simulink model "Environment"  (R2012b)
settings: Solver=FixedStepDiscrete  StartTime=0.0  StopTime=10.0  FixedStep=delta_t  RelTol=1e-3
settings Model: Creator=Kerianne  LastModifiedBy=Kerianne
settings DataIOCC: SaveFormat=Structure
settings OptimizationCC: InlineParams=on

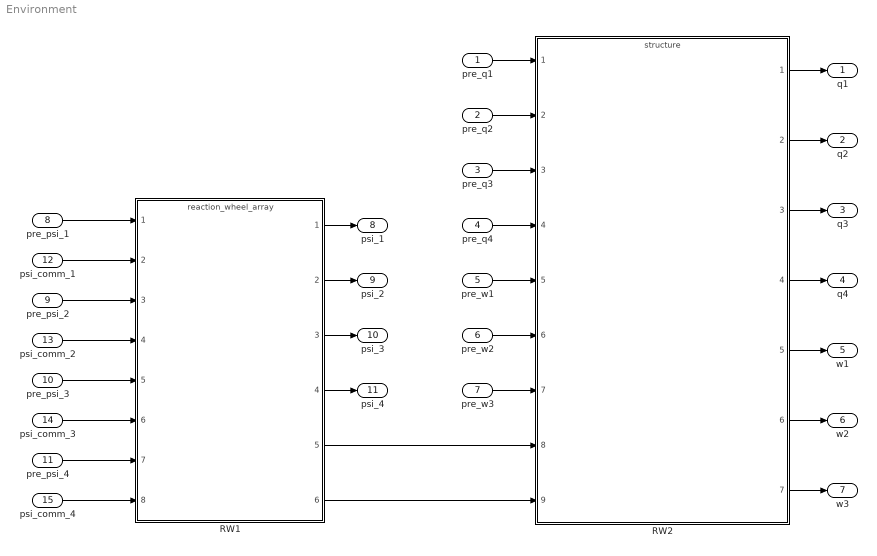
== system Environment ==
  pre_q1 : Inport
  pre_q2 : Inport  Port=2
  pre_q3 : Inport  Port=3
  pre_q4 : Inport  Port=4
  pre_w1 : Inport  Port=5
  pre_w2 : Inport  Port=6
  pre_w3 : Inport  Port=7
  pre_psi_1 : Inport  Port=8
  pre_psi_2 : Inport  Port=9
  pre_psi_3 : Inport  Port=10
  pre_psi_4 : Inport  Port=11
  "psi_comm_1 " : Inport  Port=12
  psi_comm_2 : Inport  Port=13
  psi_comm_3 : Inport  Port=14
  psi_comm_4 : Inport  Port=15
  RW1 : ModelReference  ModelNameDialog=reaction_wheel_array  SimulationMode=Normal  ModelReferenceVersion=1.14  CopyOfModelName=reaction_wheel_array  DefaultDataLogging=on
  RW2 : ModelReference  ModelNameDialog=structure  SimulationMode=Normal  ModelReferenceVersion=1.10  CopyOfModelName=structure  DefaultDataLogging=on
  q1 : Outport
  q2 : Outport  Port=2
  q3 : Outport  Port=3
  q4 : Outport  Port=4
  w1 : Outport  Port=5
  w2 : Outport  Port=6
  w3 : Outport  Port=7
  psi_1 : Outport  Port=8
  psi_2 : Outport  Port=9
  psi_3 : Outport  Port=10
  psi_4 : Outport  Port=11
  wires:
  pre_psi_1/1 -> RW1/1
  "psi_comm_1 "/1 -> RW1/2
  pre_psi_2/1 -> RW1/3
  psi_comm_2/1 -> RW1/4
  pre_psi_3/1 -> RW1/5
  psi_comm_3/1 -> RW1/6
  RW2/7 -> w3/1
  RW2/6 -> w2/1
  RW2/5 -> w1/1
  RW2/4 -> q4/1
  RW2/3 -> q3/1
  RW2/2 -> q2/1
  RW2/1 -> q1/1
  pre_w3/1 -> RW2/7
  pre_w2/1 -> RW2/6
  pre_w1/1 -> RW2/5
  pre_q4/1 -> RW2/4
  pre_q3/1 -> RW2/3
  pre_q2/1 -> RW2/2
  pre_q1/1 -> RW2/1
  RW1/3 -> psi_3/1
  RW1/2 -> psi_2/1
  RW1/1 -> psi_1/1
  RW1/6 -> RW2/9
  RW1/5 -> RW2/8
  RW1/4 -> psi_4/1
  pre_psi_4/1 -> RW1/7
  psi_comm_4/1 -> RW1/8
